simulink library "Nordic32_Lib"  (R2020b)
settings: Solver=VariableStepAuto  StartTime=0.0  StopTime=10.0  RelTol=1e-3
undefined symbols (not defined in the file or in its folder): D1, data_NREL, Delta, DiscIntNeverNeededParam, exc_Efmax, exc_Efmin, exc_Ka, exc_Ta, exc_Tb, exc_Tc, ExcData, fn, gcbh, gen_Xt, GenData, Gwind, Gwind_speed, lines, loads, mac_con, PSSData, sps_rtmsupport, time_activate_wind, trafos, wind_turbines
libraries: powerlib x18, $bdroot x13, powerlib_meascontrol x4, simulink x3, sps_avr x2, dspsigops x2, spsExcitationSystemModel x1, eeGeneralControl x1
(part 1 of 2)
settings Model: Creator=joakbj  LastModifiedBy=joakim
settings DataIOCC: ReturnWorkspaceOutputs=off
settings DebuggingCC: ArithmeticOperatorsInVariantConditions=warning
settings SFSimCC: SimUseLocalCustomCode=off  CustomCodeUndefinedFunction=UseInterfaceOnly
settings RTWCC: RTWUseLocalCustomCode=off
settings CodeAppCC: StateflowObjectComments=on

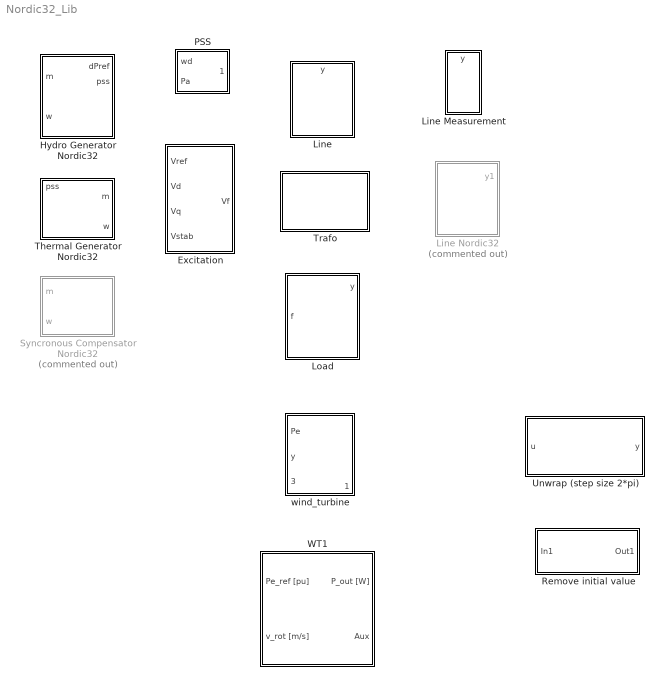
== system Nordic32_Lib ==
  Excitation : Subsystem  mask{K_a=300, sat_bounds=[0, 5]}
      mask prompts: K_a "gain"; sat_bounds "Saturation"
  Hydro Generator Nordic32 : Subsystem  mask{i=1, gen_data=GenData, pss_data=PSSData, exc_data=ExcData, ii=1, FCR_reg=tf(1), fn=fn, open_loop_on=0}
      mask prompts: i "Generator Number"; gen_data "Generator and Governor Data Table"; pss_data "PSS Data Table"; exc_data "Exciter Data Table"; ii "FCR regulator number"; FCR_reg "FCR controller transfer function"; fn "Nominal Frequency"; open_loop_on "Open loop test?"
      mask init:
      | % GenNumber = i;
      | gen_data = gen_data(i,:);
      | pss_data = pss_data(i,:);
      | exc_data = exc_data(i,:);
      | 
      | % Name to display
      | if gen_data.GenType == 1;
      |     if gen_data.GovType == 1;
      |         name = ['Hydro G', num2str(i)]; % Salient pole generator with hydro governor
      |         % Governor parameters
      |         gov_Ta = gen_data.Ta;
      |         % Gate opening limits [gmin, gmax (pu)  vgmin,vgmax(pu/s)]
      |         gov_gate= [gen_data.gMIN,  gen_data.gMAX,...
      |                   -gen_data.vgMAX, gen_data.vgMAX];
      |         % Permanent droop and regular [Rp Kp Ki Kd Td] %%% UNUSED
      | %         gov_gain = [gen_data.R, 1/gen_data.r,...
      | %                     1/(gen_data.r*gen_data.Tr),...
      | %                     0/(gen_data.r), gen_data.Tf]; 
      |         gov_num = FCR_reg.NUM{1}; % Replaces gov_gain
      |         gov_den = FCR_reg.DEN{1};
      |         gov_TW = gen_data.TW;        
      |     else
      |         name = ['erSCG', num2str(i)]; % Salient pole syncronous compensator
      |     end
      | elseif gen_data.GenType == 2;
      |     if gen_data.GovType == 0;
      |         name = ['erTG', num2str(i)]; % Round rotor generator, thermal plan no governor
      |     else
      |         name = ['erTgovG', num2str(i)]; % No Round rotor generator should have governor
      |     end
      | end
      | 
      | P = gen_data.PGEN;
      | Qmin = gen_data.QMIN;
      | Qmax = gen_data.QMAX;
      | Sb = gen_data.MBASE;
      | 
      | %% Display set power, need to adjust character length
      | set_power = ['P ', num2str(round(P,0))];
      | base_power = ['Sb ', num2str(round(Sb,0))];
      | fcr_name = ['FCR ', num2str(ii)];
      | l1 = strlength(name);
      | l2 = strlength(set_power);
      | l3 = strlength(base_power);
      | l4 = strlength(fcr_name);
      | lmax = max([l1,l2,l3,l4]);
      | 
      | for iter = 1:lmax-l1 % 
      |     name = [name, ' '];
      | end
      | for iter = 1:lmax-l2 % String with generator name has more characters
      |     set_power = [set_power, ' '];
      | end
      | for iter = 1:lmax-l3 % String with generator name has more characters
      |     base_power = [base_power, ' '];
      | end
      | for iter = 1:lmax-l4 % String with generator name has more characters
      |     fcr_name = [fcr_name, ' '];
      | end
      | 
      | name = [name;set_power;base_power;fcr_name];
      | 
      | % Generator parameters
      | gen_Pn = gen_data.MBASE; % Nominal power (MW)
      | gen_Vn = gen_data.BSKV; % Nominal voltage (kV)
      | % Reactances [Xd Xd' Xd'' Xq Xq'' Xl] (pu)
      | gen_X = [gen_data.Xd, gen_data.Xdp, gen_data.Xdpp,...
      |      gen_data.Xq, gen_data.Xqpp, gen_data.XL];
      | % Time constants [Tdo' Tdo'' Tqo''] (s)
      | gen_T = [gen_data.Td0p, gen_data.Td0pp, gen_data.Tq0pp];
      | gen_H = gen_data.H; % Inertia coefficient (s)
      | 
      | %% Governor Secondary (Frequency restoration)
      | % Ri = gen_data.Ri;
      | % Generator trafo (H)
      | % gen_Xt = gen_data.Xt*gen_Vn/(gen_Pn*2*pi*fn);
      | 
      | % gen_X = gen_X + gen_data.Xt;
      mask Display: disp(name)
  Line : Subsystem  mask{i=1, data=lines, fn=fn}
      mask prompts: i "Line Number"; data "Line Data Table"; fn "Nominal Freq"
      mask init:
      | km = data.km(i);
      | Vn = data.V(i);
      settings: PortSchema="{\"entries\":[{\"content\":{\"sides\":[{\"content\":{\"connectorIds\":[\"LConn1\",\"LConn2\",\"LConn3\"]},\"type\":\"ConnectorPlacement.EquallySpacedRectSide\",\"uuid\":\"159cc543-018e-4826-b622-a4d07c97e386\"},{\"content\":{\"connectorIds\":[\"RConn1\",\"RConn2\",\"RConn3\"],\"side\":\"RIGHT\"},\"type\":\"ConnectorPlacement.EquallySpacedRectSide\",\"uuid\":\"cb1aeae8-69bb-45ac-8689-4e8674d58501\"},{\"content\":{\"connectorIds\":[\"Out1\"],\"side\":\"TOP\"},\"type\":\"ConnectorPlacement.EquallySpacedRectSide\",\"uuid\":\"62a962af-3de7-4ff9-a859-7af1186eef9e\"}]},\"type\":\"ConnectorPlacement.EquallySpacedConnector\",\"uuid\":\"81b99b7d-1491-4204-9648-8ec0c780f157\"}],\"packageUris\":[\"http://schema.mathworks.com/mf0/Connector/19700101\"],\"version\":\"1.0\"}"
      mask Display:
      | str1 = [num2str(i)];
      | % str1 = [num2str(i)];
      | str2 = [num2str(data.from(i))];
      | str3 = [num2str(data.to(i))];
      | str4 = [num2str(data.km(i)) 'km'];
      | 
      | 
      | m = max([length(str1), length(str2), length(str3),...
      |     length(str4)]);
      | 
      | for j = length(str1):m-1
      |     str1 = [str1, ' '];
      | end
      | for j = length(str2):m-1
      |     str2 = [str2, ' '];
      | end
      | for j = length(str3):m-1
      |     str3 = [str3, ' '];
      | end
      | for j = length(str4):m-1
      |     str4 = [str4, ' '];
      | end
      | 
      | 
      | disp([str1; str2; str3; str4])
  Line Measurement : Subsystem
      settings: PortSchema="{\"entries\":[{\"content\":{\"sides\":[{\"content\":{\"connectorIds\":[\"LConn1\",\"LConn2\",\"LConn3\"]},\"type\":\"ConnectorPlacement.EquallySpacedRectSide\",\"uuid\":\"159cc543-018e-4826-b622-a4d07c97e386\"},{\"content\":{\"connectorIds\":[\"RConn1\",\"RConn2\",\"RConn3\"],\"side\":\"RIGHT\"},\"type\":\"ConnectorPlacement.EquallySpacedRectSide\",\"uuid\":\"cb1aeae8-69bb-45ac-8689-4e8674d58501\"},{\"content\":{\"connectorIds\":[\"Out1\"],\"side\":\"TOP\"},\"type\":\"ConnectorPlacement.EquallySpacedRectSide\",\"uuid\":\"62a962af-3de7-4ff9-a859-7af1186eef9e\"}]},\"type\":\"ConnectorPlacement.EquallySpacedConnector\",\"uuid\":\"81b99b7d-1491-4204-9648-8ec0c780f157\"}],\"packageUris\":[\"http://schema.mathworks.com/mf0/Connector/19700101\"],\"version\":\"1.0\"}"
      mask Display: disp(['|V|'; 'ang'; ' P '; ' Q '])
  Line Nordic32 : Subsystem  Commented=on  mask{i=1, data=lines, fn=fn}
      mask prompts: i "Line Number"; data "Line Data Table"; fn "Nominal frequency"
      mask init:
      | r = data.r(i);
      | r0 = data.r0(i);
      | l = data.l(i);
      | l0 = data.l0(i);
      | c = data.c(i);
      | c0 = data.c0(i);
      | Vn = data.V(i);
      mask Display: disp([i;data.from(i);data.to(i)])
  Load : Subsystem  mask{i=1, data=loads, fn=fn, local_freq=1}
      mask prompts: i "Load numer"; data "Load Data Table"; fn "Nominal Frequency"; local_freq "Use local frequency for loads"
      mask init:
      | data_ = data(i,:);
      | BUS = data_.BUS;
      | Vn = data_.V;
      | PL = data_.PL;
      | PL_freq = data_.PL_freq;
      | QL = data_.QL;
      | np = data_.np;
      | nq = data_.nq;
      | PSHUNT = data_.PSHUNT;
      | QSHUNT = data_.QSHUNT; % Capacitor (Negative means reactor)
      | if QSHUNT < 0
      |     QSHUNTpos = 0;
      |     QSHUNTneg = -QSHUNT;
      | else
      |     QSHUNTpos = QSHUNT;
      |     QSHUNTneg = 0;
      | end
      | 
      | %% Display active load, need to adjust character length
      | name = [num2str(BUS)];
      | strPL = ['PL ', num2str(PL)];
      | strQL = ['QL ', num2str(QL)];
      | strSH= ['SH ', num2str(QSHUNT)];
      | strV= [num2str(Vn), ' kV'];
      | l1 = strlength(name);
      | l2 = strlength(strPL);
      | l3 = strlength(strQL);
      | l4 = strlength(strSH);
      | l5 = strlength(strV);
      | lmax = max([l1,l2,l3,l4,l5]);
      | 
      | if lmax > l1
      | for iter = 1:lmax-l1 % String with set power has more characters
      |     name = [name, ' '];
      | end
      | end
      | if lmax >l2
      | for iter = 1:lmax-l2 % String with generator name has more characters
      |     strPL = [strPL, ' '];
      | end
      | end
      | if lmax > l3
      | for iter = 1:lmax-l3 % String with generator name has more characters
      |     strQL = [strQL, ' '];
      | end
      | end
      | if lmax > l4
      | for iter = 1:lmax-l4 % String with generator name has more characters
      |     strSH = [strSH, ' '];
      | end
      | end
      | if lmax > l5
      | for iter = 1:lmax-l5 % String with generator name has more characters
      |     strV = [strV, ' '];
      | end
      | end
      | 
      | name = [name;strPL;strQL;strSH;strV];
      mask Display: disp([name])
  "PSS " : Subsystem  mask(Power System Stabilizer, Nordic32){Tpss=[0, 0, 0, 0], Kpss=0, sat_bounds=[-0.05, 0.05], Tw=4.5, Tf=0.05}
      mask prompts: Tpss "time constants [T1, T2, T3, T4]"; Kpss "gain"; sat_bounds "saturation"; Tw "washout"; Tf "low_pass"
      mask help: This block implements a Power System Stabilizer as defined in Nordic32 CIGRE report
      mask init:
      | T1 = Tpss(1);
      | T2 = Tpss(2);
      | T3 = Tpss(3);
      | T4 = Tpss(4);
      | VMIN = sat_bounds(1);
      | VMAX = sat_bounds(2);
  Remove initial value : Subsystem
  Syncronous Compensator Nordic32 : Subsystem  Commented=on  mask{i=13, gen_data=GenData, pss_data=PSSData, exc_data=ExcData, fn=fn}
      mask prompts: i "Generator Number"; gen_data "Generator and Governor Data Table"; pss_data "PSS Data Table"; exc_data "Exciter Data Table"; fn "Nominal Frequency"
      mask init:
      | % GenNumber = i;
      | gen_data = gen_data(i,:);
      | pss_data = pss_data(i,:);
      | exc_data = exc_data(i,:);
      | 
      | % Name to display
      | if gen_data.GenType == 1;
      |     if gen_data.GovType == 1;
      |         name = ['erHgovG', num2str(i)]; % Salient pole generator with hydro governor
      |         % Governor parameters
      |         gov_Ta = gen_data.Ta;
      |         % Gate opening limits [gmin, gmax (pu)  vgmin,vgmax(pu/s)]
      |         gov_gate= [gen_data.gMIN,  gen_data.gMAX,...
      |                   -gen_data.vgMAX, gen_data.vgMAX];
      |         % Permanent droop and regular [Rp Kp Ki Kd Td]
      |         gov_gain = [gen_data.R, 1/gen_data.r,...
      |                     1/(gen_data.r*gen_data.Tr),...
      |                     0, gen_data.Tf];
      |         gov_TW = gen_data.TW;        
      |     else
      |         name = ['SCG', num2str(i)]; % Salient pole syncronous compensator
      |     end
      | elseif gen_data.GenType == 2;
      |     if gen_data.GovType == 0;
      |         name = ['erTG', num2str(i)]; % Round rotor generator, thermal plan no governor
      |     else
      |         name = ['erTgovG', num2str(i)]; % No Round rotor generator should have governor
      |     end
      | end
      | 
      | P = gen_data.PGEN;
      | Qmin = gen_data.QMIN;
      | Qmax = gen_data.QMAX;
      | Sb = gen_data.MBASE;
      | 
      | %% Display set power, need to adjust character length
      | set_power = ['P ', num2str(P)];
      | base_power = ['Sb ', num2str(Sb)];
      | l1 = strlength(name);
      | l2 = strlength(set_power);
      | l3 = strlength(base_power);
      | lmax = max([l1,l2,l3]);
      | 
      | for iter = 1:lmax-l1 % 
      |     name = [name, ' '];
      | end
      | for iter = 1:lmax-l2 % String with generator name has more characters
      |     set_power = [set_power, ' '];
      | end
      | for iter = 1:lmax-l3 % String with generator name has more characters
      |     base_power = [base_power, ' '];
      | end
      | 
      | name = [name;set_power;base_power];
      | 
      | % Generator parameters
      | gen_Pn = gen_data.MBASE; % Nominal power (MW)
      | gen_Vn = gen_data.BSKV; % Nominal voltage (kV)
      | % Reactances [Xd Xd' Xd'' Xq Xq'' Xl] (pu)
      | gen_X = [gen_data.Xd, gen_data.Xdp, gen_data.Xdpp,...
      |      gen_data.Xq, gen_data.Xqpp, gen_data.XL];
      | % Time constants [Tdo' Tdo'' Tqo''] (s)
      | gen_T = [gen_data.Td0p, gen_data.Td0pp, gen_data.Tq0pp];
      | gen_H = gen_data.H; % Inertia coefficient (s)
      | % Generator trafo (H)
      | % gen_Xt = gen_data.Xt*gen_Vn/(gen_Pn*2*pi*fn);
      | % gen_X = gen_X + gen_data.Xt;
      | 
      | % Exciter parameters
      | exc_Ka = exc_data.K;
      | exc_Ta = exc_data.TC;
      | exc_Tb = exc_data.TAdivbyTB*exc_data.TB;
      | exc_Tc = exc_data.TB;
      | exc_Efmin = exc_data.MIN;
      | exc_Efmax = exc_data.MAX;
      | 
      | % PSS
      | PSSNumber = pss_data.PSSNumber;
      mask Display: disp(name)
  Thermal Generator Nordic32 : Subsystem  mask{i=4, gen_data=GenData, pss_data=PSSData, exc_data=ExcData, fn=fn}
      mask prompts: i "Generator Number"; gen_data "Generator and Governor Data Table"; pss_data "PSS Data Table"; exc_data "Exciter Data Table"; fn "Nominal Frequency"
      mask init:
      | % GenNumber = i;
      | gen_data = gen_data(i,:);
      | pss_data = pss_data(i,:);
      | exc_data = exc_data(i,:);
      | 
      | % Name to display
      | if gen_data.GenType == 1;
      |     if gen_data.GovType == 1;
      |          name = ['erHgovG', num2str(i)]; % Salient pole generator with hydro governor
      | %         Governor parameters
      | %         gov_Ta = gen_data.Ta;
      | %         Gate opening limits [gmin, gmax (pu)  vgmin,vgmax(pu/s)]
      | %         gov_gate= [gen_data.gMIN,  gen_data.gMAX,...
      | %                   -gen_data.vgMAX, gen_data.vgMAX];
      | %         Permanent droop and regular [Rp Kp Ki Kd Td]
      | %         gov_gain = [gen_data.R, 1/gen_data.r,...
      | %                     1/(gen_data.r*gen_data.Tr),...
      | %                     0, gen_data.Tf];
      | %         gov_TW = gen_data.TW;        
      |     else
      |         name = ['erSCG', num2str(i)]; % Salient pole syncronous compensator
      |     end
      | elseif gen_data.GenType == 2;
      |     if gen_data.GovType == 0;
      |         name = ['Th G', num2str(i)]; % Round rotor generator, thermal plan no governor
      |     else
      |         name = ['erTgovG', num2str(i)]; % No Round rotor generator should have governor
      |     end
      | end
      | 
      | P = gen_data.PGEN;
      | Qmin = gen_data.QMIN;
      | Qmax = gen_data.QMAX;
      | Sb = gen_data.MBASE;
      | 
      | %% Display set power, need to adjust character length
      | set_power = ['P ', num2str(round(P,0))];
      | base_power = ['Sb ', num2str(round(Sb,0))];
      | l1 = strlength(name);
      | l2 = strlength(set_power);
      | l3 = strlength(base_power);
      | lmax = max([l1,l2,l3]);
      | 
      | for iter = 1:lmax-l1 % 
      |     name = [name, ' '];
      | end
      | for iter = 1:lmax-l2 % String with generator name has more characters
      |     set_power = [set_power, ' '];
      | end
      | for iter = 1:lmax-l3 % String with generator name has more characters
      |     base_power = [base_power, ' '];
      | end
      | 
      | name = [name;set_power;base_power];
      | 
      | % Generator parameters
      | gen_Pn = gen_data.MBASE; % Nominal power (MW)
      | gen_Vn = gen_data.BSKV; % Nominal voltage (kV)
      | % Reactances [Xd Xd' Xd'' Xq Xq' Xq'' Xl] (pu)
      | gen_X = [gen_data.Xd, gen_data.Xdp, gen_data.Xdpp,...
      |          gen_data.Xq, gen_data.Xqp, gen_data.Xqpp, gen_data.XL];
      | % Time constants [Tdo' Tdo'' Tqo' Tqo''] (s)
      | gen_T = [gen_data.Td0p, gen_data.Td0pp,...
      |          gen_data.Tq0p, gen_data.Tq0pp];
      | gen_H = gen_data.H; % Inertia coefficient (s)
      | % Generator trafo (H)
      | gen_Xt = gen_data.Xt*gen_Vn/(gen_Pn*2*pi*fn);
      | % gen_X = gen_X + gen_data.Xt;
      mask Display: disp(name)
  Trafo : Subsystem  mask{i=2, data=trafos, fn=fn}
      mask prompts: i "Trafo number"; data "Trafo Data Table"; fn "Nominal frequency"
      mask init:
      | V1 = data.V1(i);
      | V2 = data.V2(i);
      | L2 = data.L2(i);
      | ratio = data.ratio(i);
      | Sbase = data.Sbase(i);
      mask Display:
      | str1 = [num2str(i)];
      | % str1 = [num2str(i)];
      | str2 = [num2str(data.from(i)), ': ', num2str(data.V1(i)), 'kV'];
      | str3 = [num2str(data.to(i)), ': ', num2str(data.V2(i)), 'kV'];
      | str4 = ['x=',  num2str(data.L2(i)) 'pu'];
      | str5 = ['Sb=', num2str(data.Sbase(i))];
      | 
      | m = max([length(str1), length(str2), length(str3),...
      |     length(str4),length(str5)]);
      | 
      | for j = length(str1):m-1
      |     str1 = [str1, ' '];
      | end
      | for j = length(str2):m-1
      |     str2 = [str2, ' '];
      | end
      | for j = length(str3):m-1
      |     str3 = [str3, ' '];
      | end
      | for j = length(str4):m-1
      |     str4 = [str4, ' '];
      | end
      | for j = length(str5):m-1
      |     str5 = [str5, ' '];
      | end
      | 
      | disp([str1; str2; str3; str4; str5])
  Unwrap (step size 2*pi) : Subsystem
  WT1 : Subsystem  mask(Wind Turbine){w_gen_ini=data_NREL.w_initial, beta_ini=0, auto=off, torq_ini=data_NREL.torque_initial, data=data_NREL}
      mask prompts: w_gen_ini "Initial generator velocity  [rad/s]"; beta_ini "Initial blade pitch [degrees]"; auto "Auto initial torque"; torq_ini "Initial generator torque"; data "Data NREL Wind turbine"
      mask help: NREL 5MW Virtual Turbine
      mask init:
      | %l=load(file);
      | env=data.env;
      | wt=data.wt;
      | wt.ctrl.gen.ini=w_gen_ini;
      | ctrl=data.ctrl;
      | 
      | if(auto)
      |     wt.ctrl.torq.ini=min(interp1(wt.ctrl.torq.wg,wt.ctrl.torq.M,w_gen_ini,'spline'),wt.ctrl.torq.lim);
      | else
      |     wt.ctrl.torq.ini=torq_ini;
      | end
      | 
      | wt.pitch.ini=beta_ini;
      | wt.ctrl.pitch.ini=beta_ini;
      | wt.gen.torq.ini=wt.ctrl.torq.ini;
      | wt.gen.ini=w_gen_ini;
      | wt.rotor.ini=w_gen_ini/wt.gen.N;
      mask Display:
      | image(imread('NREL.png'))
      | 
      | port_label('output',1,'P [W]')
      | % port_label('output',2,'CT')
      | % port_label('output',3,'w_gen [rad/s]')
      | % port_label('output',4,'v_nac [m/s]')
      | % port_label('output',5,'pitch [deg]')
      | % port_label('output',6,'M_shaft [Nm]')
      | % port_label('output',7,'M_tow [Nm]')
      | % port_label('output',8,'Aux')
      | port_label('output',2,'Aux')
      | 
      | port_label('input',1,'P/P_opt [pu]')
      | port_label('input',2,'v_rot [m/s]')
      | % port_label('input',3,'v_nac [m/s]')
  wind_turbine : Subsystem  mask{i=1, data=wind_turbines, data_NREL=data_NREL, fn=fn, time_activate_wind=time_activate_wind, Gwind=Gwind, Gwind_speed=Gwind_speed, FCR=tf(1)}
      mask prompts: i "Turbine number"; data "Wind Turbine Load Flow Data"; data_NREL "Wind Model Data"; fn "Nominal freqeuncy"; time_activate_wind "Activate wind turbine model at time:"; Gwind "Linear model, Pref -> Pe"; Gwind_speed "Linear model, Pref -> speed"; FCR "FCR, y -> Pref"
      mask init:
      | data = data(i,:); 
      | 
      | Vn = data.BSKV;
      | MBASE = data.MBASE;
      | POPT = data.POPT;
      | 
      | if iscell(data_NREL)
      |     data_NREL = data_NREL{i};
      | end
      | 
      | strWindSpeed = ['v = ', num2str(data.V_WIND)];
      | strWind = ['wind(',num2str(i),') ' num2str(MBASE)];
      | strWindOpt = ['Popt ', num2str(round(POPT,0))];
      | strV= [num2str(Vn), ' kV'];
      | 
      | l1 = strlength(strWind);
      | l2 = strlength(strWindOpt);
      | l3 = strlength(strV);
      | l4 = strlength(strWindSpeed);
      | lmax = max([l1,l2,l3,l4]);
      | 
      | if lmax > l1
      | for iter = 1:lmax-l1 % String with generator name has more characters
      |     strWind = [strWind, ' '];
      | end
      | end
      | if lmax > l2
      | for iter = 1:lmax-l2 % String with generator name has more characters
      |     strWindOpt = [strWindOpt, ' '];
      | end
      | end
      | if lmax > l3
      | for iter = 1:lmax-l3 % String with generator name has more characters
      |     strV = [strV, ' '];
      | end
      | end
      | if lmax > l4
      | for iter = 1:lmax-l4 % String with generator name has more characters
      |     strWindSpeed = [strWindSpeed, ' '];
      | end
      | end
      | 
      | name = [strWindSpeed;strWind;strWindOpt;strV];
      settings: PortSchema="{\"entries\":[{\"content\":{\"sides\":[{\"content\":{\"connectorIds\":[\"LConn1\",\"LConn2\",\"LConn3\",\"In1\"]},\"type\":\"ConnectorPlacement.EquallySpacedRectSide\",\"uuid\":\"48445341-a685-4506-9ec8-e376e0c1b939\"},{\"content\":{\"connectorIds\":[\"Out1\",\"Out2\",\"Out3\"],\"side\":\"RIGHT\"},\"type\":\"ConnectorPlacement.EquallySpacedRectSide\",\"uuid\":\"cf3481ef-9523-4ae9-af94-5a03f7da080c\"},{\"content\":{\"connectorIds\":[],\"side\":\"TOP\"},\"type\":\"ConnectorPlacement.EquallySpacedRectSide\",\"uuid\":\"cf4caa18-6df0-400d-a59e-8b335f5a193c\"}]},\"type\":\"ConnectorPlacement.EquallySpacedConnector\",\"uuid\":\"872d10b1-fdd8-4789-878b-9f44ab3824be\"}],\"packageUris\":[\"http://schema.mathworks.com/mf0/Connector/19700101\"],\"version\":\"1.0\"}"
      mask Display: disp([name])

== system Nordic32_Lib/Excitation ==
  Vref : Inport
  Vd : Inport  Port=2
  Vq : Inport  Port=3
  Vstab : Inport  Port=4
  EXCITATION Nordic32 : sps_avr/Excitation System  Commented=on  tr=0.02  reg=[exc_Ka, exc_Ta]  exc=[ 1, 0 ]  tgr=[exc_Tb, exc_Tc]  damp=[ 1e-3 0.1]*0  sat=[ 0, 0 ]  lim=[exc_Efmin, exc_Efmax, 0 ]  v0=[1,1.07168]
      settings: SourceProductBaseCode=PS
  Excitation Standard : Subsystem  DialogController=POWERSYS.PowerSysDialog  LoadFcn=sps_rtmsupport('LoadFcn', gcbh);  StartFcn=sps_rtmsupport('StartFcn', gcbh);  StopFcn=sps_rtmsupport('StopFcn', gcbh);  mask(Excitation System){tr=20e-3, reg=[ K_a, 0.001 ], exc=[ 1, 0 ], tgr=[ 0, 0 ], damp=[ 0.001, 0.1 ], sat=[ 0, 0 ], lim=[sat_bounds(1), sat_bounds(2), 0 ], v0=[1.0  1.28]}
      mask prompts: tr "Low-pass filter time constant Tr(s):"; reg "Regulator gain and time constant [ Ka()  Ta(s) ]:"; exc "Exciter  [ Ke()  Te(s) ]:"; tgr "Transient gain reduction [ Tb(s)  Tc(s) ]:"; damp "Damping filter gain and time constant  [ Kf()  Tf(s)  ]:"; sat "Field saturation parameters [ A, B ]:"; lim "Regulator output limits and gain [ Efmin, Efmax (pu), Kp() ]:"; v0 "Initial values of terminal voltage  and field voltage [ Vt0 (pu) Vf0(pu) ] :"
      mask help:
      | Implements an IEEE type 1 synchronous machine voltage regulator combined
      | to an exciter.
      |
      | The output of the block is the field voltage vfd, in pu,  to be applied to the Vf
      | Simulink input of a Synchronous Machine block.
      |
      | Connect the Vd and Vq measurements signals of the Synchronous Machine block
      | (signals 9 and 10)  to  the Vd and Vq inputs of the Excitation System block.
      mask init:
      | block = gcb;
      | [Ts, WantBlockChoice,MaskType, ka,ta,ke,te,tb,tc,kf,tf,efmin,efmax,kp,a,b] = powericon('ExcitationSystemInit',block,-2,reg,exc,tgr,damp,lim,sat);
      | powericon('SetInternalModels','set',block,WantBlockChoice);
      settings: CopyFcn=sps_rtmsupport('CopyFcn', gcbh);  DeleteFcn=sps_rtmsupport('DeleteFcn', gcbh);  UndoDeleteFcn=sps_rtmsupport('UndoDeleteFcn', gcbh);  ModelCloseFcn=sps_rtmsupport('ModelCloseFcn', gcbh);  PreSaveFcn=sps_rtmsupport('PreSaveFcn', gcbh);  PostSaveFcn=sps_rtmsupport('PostSaveFcn', gcbh);  NameChangeFcn=sps_rtmsupport('NameChangeFcn', gcbh);  PreCopyFcn=sps_rtmsupport('PreCopyFcn', gcbh);  OpenFcn=sps_rtmsupport('OpenFcn', gcbh, []);  CloseFcn=sps_rtmsupport('CloseFcn', gcbh);  PreDeleteFcn=sps_rtmsupport('PreDeleteFcn', gcbh);
      mask Help: helpview(psbhelp);
      mask Display: disp('')
  Vf : Outport
  wires:
  Excitation Standard/1(Vf) -> Vf/1
  Vq/1 -> Excitation Standard/3(Vq)
  Vd/1 -> Excitation Standard/2(Vd)
  Vstab/1 -> Excitation Standard/4(Vstab)
  Vref/1 -> Excitation Standard/1(Vref)

== system Nordic32_Lib/Hydro Generator Nordic32 ==
  dPref : Inport
  pss : Inport  Port=2
  " MBASE MVA 400 kV-400 kV" : powerlib/Elements/Three-Phase Transformer (Two Windings)  Winding1Connection=Delta (D1)  Winding2Connection=Yg  CoreType=Three single-phase transformers  SetSaturation=off  Hysteresis=off  DataFile='hysteresis'  SetInitialFlux=off  Measurements=None  UNITS=pu  NominalPower="[ gen_Pn*1e6  fn ]"  Winding1="[ gen_Vn*1e3  1e-6   0  ]"  Winding2="[ gen_Vn*1e3   1e-6  gen_data.Xt ]"  Rm=500  Lm=500  L0=0.5  Saturation="[ 0,0  ;  0.005,1.2  ;  1.0,1.4 ]"  InitialFluxes=[ 0.8 , -0.8 , 0.7 ]  BreakLoop=off  DiscreteSolver=Trapezoidal iterative  DataType=off  TransfoNumber=0
  Bus Selector : BusSelector  OutputSignals="Rotor speed  wm  (pu)"
  Generator : powerlib/Machines/Synchronous Machine pu Standard  PresetModel=No  MechanicalLoad=Mechanical power Pm  ShowDetailedParameters=on  RotorType=Salient-pole  Units=per unit standard parameters  MeasurementBus=off  NominalParameters=[gen_Pn*1e6, gen_Vn*1e3, fn]  Reactances1="[mac_con(1,6:8)  mac_con(1,11:13)  mac_con(1,4)]"  Reactances2=gen_X  dAxisTimeConstants=Open-circuit  qAxisTimeConstants=Open-circuit  TimeConstants1=gen_T  TimeConstants2="[mac_con(1,9:10)  mac_con(1,14:15)]"  TimeConstants3=[]  TimeConstants4=[]  TimeConstants5=[ 1.01, 0.053, 0.1 ]  TimeConstants6=[]  TimeConstants7=gen_T  TimeConstants8=[]  StatorResistance=[1e-9]  Mechanical="[gen_H 0  4]"  PolePairs=4  InitialConditions=[0 -53.3817 1.03438 1.03438 1.03438 11.5505 -108.45 131.55 1.07168]  SetSaturation=off  Saturation=[0.6404,0.7127,0.8441,0.9214,0.9956,1.082,1.19,1.316,1.457;0.7,0.7698,0.8872,0.9466,0.9969,1.046,1.1,1.151,1.201]  LoadFlowParameters=[1 1000000000 0 0 0]  TsPowergui=0  TsBlock=-1  IterativeModel=Forward Euler  IterativeDiscreteModel=Trapezoidal non iterative  BusType=PV  Pref=P*1e6  Qref=0  Qmin=Qmin*1e6  Qmax=Qmax*1e6  PLF=0  QLF=0
      settings: AttributesFormatString=\n\n
  Pref : Constant
  Turbine & Regulators : Subsystem
  Vref : Constant
  A : PMIOPort  Side=Left
  B : PMIOPort  Port=2  Side=Left
  C : PMIOPort  Port=3  Side=Left
  m : Outport  VectorParamsAs1DForOutWhenUnconnected=off
  w : Outport  Port=2  VectorParamsAs1DForOutWhenUnconnected=off
  wires:
  Turbine & Regulators/2(Vf) -> Generator/2
  Generator/1 -> Turbine & Regulators/1(m)
  Vref/1 -> Turbine & Regulators/3(Vref)
  Turbine & Regulators/3(Signals) -> m/1, Bus Selector/1
  Turbine & Regulators/1(Pm) -> Generator/1
  Pref/1 -> Turbine & Regulators/2(Pref)
  Bus Selector/1 -> w/1  "<Rotor speed  wm  (pu)>"
  dPref/1 -> Turbine & Regulators/4(open_loop)
  pss/1 -> Turbine & Regulators/5(d_Vstab)
  connections:
  " MBASE MVA 400 kV-400 kV"/LConn1 -- Generator/RConn1
  " MBASE MVA 400 kV-400 kV"/LConn2 -- Generator/RConn2
  " MBASE MVA 400 kV-400 kV"/LConn3 -- Generator/RConn3
  " MBASE MVA 400 kV-400 kV"/RConn1 -- A/RConn1
  B/RConn1 -- " MBASE MVA 400 kV-400 kV"/RConn2
  C/RConn1 -- " MBASE MVA 400 kV-400 kV"/RConn3

== system Nordic32_Lib/Line ==
  Bus Creator : BusCreator  Inputs=2
  Distributed Parameters Line : powerlib/Elements/Distributed Parameters Line  Phases=3  Length=km  Frequency=fn  Resistance=[0.01273 0.3864]  Inductance="[0.9337e-3  4.1264e-3]"  Capacitance=[12.74e-9 7.751e-9]  x1=[0 0 0 0; 0.0001244 0 0 0; 0.0002488 0 0 0; 0.0003733 0 0 0; 0.0004977 0 0 0; 0.0006221 0 0 0]  x2=[0 0 0 0; 0.0001244 0 0 0; 0.0002488 0 0 0; 0.0003733 0 0 0; 0.0004977 0 0 0; 0.0006221 0 0 0]  x3=[0 0 0 0; 0.0001244 0 0 0; 0.0002488 0 0 0; 0.0003733 0 0 0; 0.0004977 0 0 0; 0.0006221 0 0 0]  x4=[0 0 0 0; 0.0001244 0 0 0; 0.0002488 0 0 0; 0.0003733 0 0 0; 0.0004977 0 0 0; 0.0006221 0 0 0]  x5=0  V1=ones(3,3)  V2=ones(3,3)  I1=ones(3,3)  I2=ones(3,3)  nHarmo=1  Measurements=None  Decoupling=off  VsMag0=0  VrMag0=0  VsAngle0=0  VrAngle0=0  IsMag0=0  IrMag0=0  IsAngle0=0  IrAngle0=0
  Line Measurement : $bdroot/Line  Measurement  SystemSampleTime=-1  VariantActivationTime=update diagram  Latency=0  AutoFrameSizeCalculation=off
      settings: PortSchema="{\"entries\":[{\"content\":{\"sides\":[{\"content\":{\"connectorIds\":[\"LConn1\",\"LConn2\",\"LConn3\"]},\"type\":\"ConnectorPlacement.EquallySpacedRectSide\",\"uuid\":\"159cc543-018e-4826-b622-a4d07c97e386\"},{\"content\":{\"connectorIds\":[\"RConn1\",\"RConn2\",\"RConn3\"],\"side\":\"RIGHT\"},\"type\":\"ConnectorPlacement.EquallySpacedRectSide\",\"uuid\":\"cb1aeae8-69bb-45ac-8689-4e8674d58501\"},{\"content\":{\"connectorIds\":[\"Out1\"],\"side\":\"TOP\"},\"type\":\"ConnectorPlacement.EquallySpacedRectSide\",\"uuid\":\"62a962af-3de7-4ff9-a859-7af1186eef9e\"}]},\"type\":\"ConnectorPlacement.EquallySpacedConnector\",\"uuid\":\"81b99b7d-1491-4204-9648-8ec0c780f157\"}],\"packageUris\":[\"http://schema.mathworks.com/mf0/Connector/19700101\"],\"version\":\"1.0\"}"
  Line Measurement1 : $bdroot/Line  Measurement  SystemSampleTime=-1  VariantActivationTime=update diagram  Latency=0  AutoFrameSizeCalculation=off
      settings: PortSchema="{\"entries\":[{\"content\":{\"sides\":[{\"content\":{\"connectorIds\":[\"LConn1\",\"LConn2\",\"LConn3\"]},\"type\":\"ConnectorPlacement.EquallySpacedRectSide\",\"uuid\":\"159cc543-018e-4826-b622-a4d07c97e386\"},{\"content\":{\"connectorIds\":[\"RConn1\",\"RConn2\",\"RConn3\"],\"side\":\"RIGHT\"},\"type\":\"ConnectorPlacement.EquallySpacedRectSide\",\"uuid\":\"cb1aeae8-69bb-45ac-8689-4e8674d58501\"},{\"content\":{\"connectorIds\":[\"Out1\"],\"side\":\"TOP\"},\"type\":\"ConnectorPlacement.EquallySpacedRectSide\",\"uuid\":\"62a962af-3de7-4ff9-a859-7af1186eef9e\"}]},\"type\":\"ConnectorPlacement.EquallySpacedConnector\",\"uuid\":\"81b99b7d-1491-4204-9648-8ec0c780f157\"}],\"packageUris\":[\"http://schema.mathworks.com/mf0/Connector/19700101\"],\"version\":\"1.0\"}"
  A : PMIOPort  Side=Left
  B : PMIOPort  Port=2  Side=Left
  C : PMIOPort  Port=3  Side=Left
  a : PMIOPort  Port=4  Side=Right
  b : PMIOPort  Port=5  Side=Right
  c : PMIOPort  Port=6  Side=Right
  y : Outport
  wires:
  Line Measurement/1 -> Bus Creator/1
  Line Measurement1/1 -> Bus Creator/2
  Bus Creator/1 -> y/1
  connections:
  Line Measurement/LConn1 -- A/RConn1
  B/RConn1 -- Line Measurement/LConn2
  C/RConn1 -- Line Measurement/LConn3
  Distributed Parameters Line/LConn1 -- Line Measurement/RConn1
  Distributed Parameters Line/LConn2 -- Line Measurement/RConn2
  Distributed Parameters Line/LConn3 -- Line Measurement/RConn3
  Distributed Parameters Line/RConn3 -- Line Measurement1/LConn3
  Line Measurement1/RConn3 -- c/RConn1
  Line Measurement1/RConn2 -- b/RConn1
  Distributed Parameters Line/RConn2 -- Line Measurement1/LConn2
  Distributed Parameters Line/RConn1 -- Line Measurement1/LConn1
  Line Measurement1/RConn1 -- a/RConn1

== system Nordic32_Lib/Line Measurement ==
  Bus Creator : BusCreator  Inputs=4
  Gain : Gain  Gain=pi/180
  Gain1 : Gain  Gain=180/pi
  "Power (3ph, Phasor)" : powerlib_meascontrol/Measurements/Power (3ph, Phasor)
      settings: SourceProductBaseCode=PS
  Sequence Analyzer (Phasor) : powerlib_meascontrol/Measurements/Sequence Analyzer (Phasor)  seq=Positive
      settings: SourceProductBaseCode=PS
  Three-Phase V-I Measurement : powerlib/Measurements/Three-Phase V-I Measurement  VoltageMeasurement=phase-to-ground  SetLabelV=off  LabelV=Vabc  Vpu=off  VpuLL=off  CurrentMeasurement=yes  SetLabelI=off  LabelI=Iabc  Ipu=off  Pbase=1e6  Vbase=400e3  OutputType=Complex  PhasorSimulation=off  PSBequivalent=0
  Unwrap pi deg : dspsigops/Unwrap  tol=pi  InputProcessing=Columns as channels (frame based)  running=off
  A : PMIOPort  Side=Left
  B : PMIOPort  Port=2  Side=Left
  C : PMIOPort  Port=3  Side=Left
  a : PMIOPort  Port=4  Side=Right
  b : PMIOPort  Port=5  Side=Right
  c : PMIOPort  Port=6  Side=Right
  y : Outport
  wires:
  "Power (3ph, Phasor)"/2 -> Bus Creator/4  "Q"
  Three-Phase V-I Measurement/2 -> "Power (3ph, Phasor)"/2
  Three-Phase V-I Measurement/1 -> Sequence Analyzer (Phasor)/1, "Power (3ph, Phasor)"/1
  Sequence Analyzer (Phasor)/1 -> Bus Creator/1  "V"
  Unwrap pi deg/1 -> Gain1/1  "ang"
  Bus Creator/1 -> y/1
  "Power (3ph, Phasor)"/1 -> Bus Creator/3  "P"
  Sequence Analyzer (Phasor)/2 -> Gain/1  "ang"
  Gain/1 -> Unwrap pi deg/1
  Gain1/1 -> Bus Creator/2  "ang"
  connections:
  Three-Phase V-I Measurement/RConn1 -- a/RConn1
  Three-Phase V-I Measurement/LConn3 -- C/RConn1
  Three-Phase V-I Measurement/RConn3 -- c/RConn1
  Three-Phase V-I Measurement/LConn2 -- B/RConn1
  Three-Phase V-I Measurement/LConn1 -- A/RConn1
  Three-Phase V-I Measurement/RConn2 -- b/RConn1

== system Nordic32_Lib/Line Nordic32 ==
  25km Area 1 : powerlib/Elements/Three-Phase PI Section Line  LConnTagsString=a|b|c  RConnTagsString=A|B|C  Length=1  Frequency=fn  Resistances=[r r0]  Inductances=[l l0]  Capacitances=[c c0]
  Line Measurement : $bdroot/Line  Measurement  SystemSampleTime=-1  VariantActivationTime=update diagram  Latency=0  AutoFrameSizeCalculation=off
      settings: PortSchema="{\"entries\":[{\"content\":{\"sides\":[{\"content\":{\"connectorIds\":[\"LConn1\",\"LConn2\",\"LConn3\"]},\"type\":\"ConnectorPlacement.EquallySpacedRectSide\",\"uuid\":\"159cc543-018e-4826-b622-a4d07c97e386\"},{\"content\":{\"connectorIds\":[\"RConn1\",\"RConn2\",\"RConn3\"],\"side\":\"RIGHT\"},\"type\":\"ConnectorPlacement.EquallySpacedRectSide\",\"uuid\":\"cb1aeae8-69bb-45ac-8689-4e8674d58501\"},{\"content\":{\"connectorIds\":[\"Out1\"],\"side\":\"TOP\"},\"type\":\"ConnectorPlacement.EquallySpacedRectSide\",\"uuid\":\"62a962af-3de7-4ff9-a859-7af1186eef9e\"}]},\"type\":\"ConnectorPlacement.EquallySpacedConnector\",\"uuid\":\"81b99b7d-1491-4204-9648-8ec0c780f157\"}],\"packageUris\":[\"http://schema.mathworks.com/mf0/Connector/19700101\"],\"version\":\"1.0\"}"
  Line Measurement1 : $bdroot/Line  Measurement  SystemSampleTime=-1  VariantActivationTime=update diagram  Latency=0  AutoFrameSizeCalculation=off
      settings: PortSchema="{\"entries\":[{\"content\":{\"sides\":[{\"content\":{\"connectorIds\":[\"LConn1\",\"LConn2\",\"LConn3\"]},\"type\":\"ConnectorPlacement.EquallySpacedRectSide\",\"uuid\":\"159cc543-018e-4826-b622-a4d07c97e386\"},{\"content\":{\"connectorIds\":[\"RConn1\",\"RConn2\",\"RConn3\"],\"side\":\"RIGHT\"},\"type\":\"ConnectorPlacement.EquallySpacedRectSide\",\"uuid\":\"cb1aeae8-69bb-45ac-8689-4e8674d58501\"},{\"content\":{\"connectorIds\":[\"Out1\"],\"side\":\"TOP\"},\"type\":\"ConnectorPlacement.EquallySpacedRectSide\",\"uuid\":\"62a962af-3de7-4ff9-a859-7af1186eef9e\"}]},\"type\":\"ConnectorPlacement.EquallySpacedConnector\",\"uuid\":\"81b99b7d-1491-4204-9648-8ec0c780f157\"}],\"packageUris\":[\"http://schema.mathworks.com/mf0/Connector/19700101\"],\"version\":\"1.0\"}"
  A : PMIOPort  Side=Left
  a : PMIOPort  Port=2  Side=Right
  B : PMIOPort  Port=3  Side=Left
  b : PMIOPort  Port=4  Side=Right
  C : PMIOPort  Port=5  Side=Left
  c : PMIOPort  Port=6  Side=Right
  y1 : Outport
  wires:
  Line Measurement/1 -> y1/1
  connections:
  Line Measurement/LConn1 -- A/RConn1
  B/RConn1 -- Line Measurement/LConn2
  C/RConn1 -- Line Measurement/LConn3
  Line Measurement/RConn1 -- 25km Area 1/LConn1
  Line Measurement/RConn2 -- 25km Area 1/LConn2
  Line Measurement/RConn3 -- 25km Area 1/LConn3
  Line Measurement1/LConn3 -- 25km Area 1/RConn3
  Line Measurement1/RConn3 -- c/RConn1
  Line Measurement1/RConn2 -- b/RConn1
  25km Area 1/RConn2 -- Line Measurement1/LConn2
  25km Area 1/RConn1 -- Line Measurement1/LConn1
  Line Measurement1/RConn1 -- a/RConn1

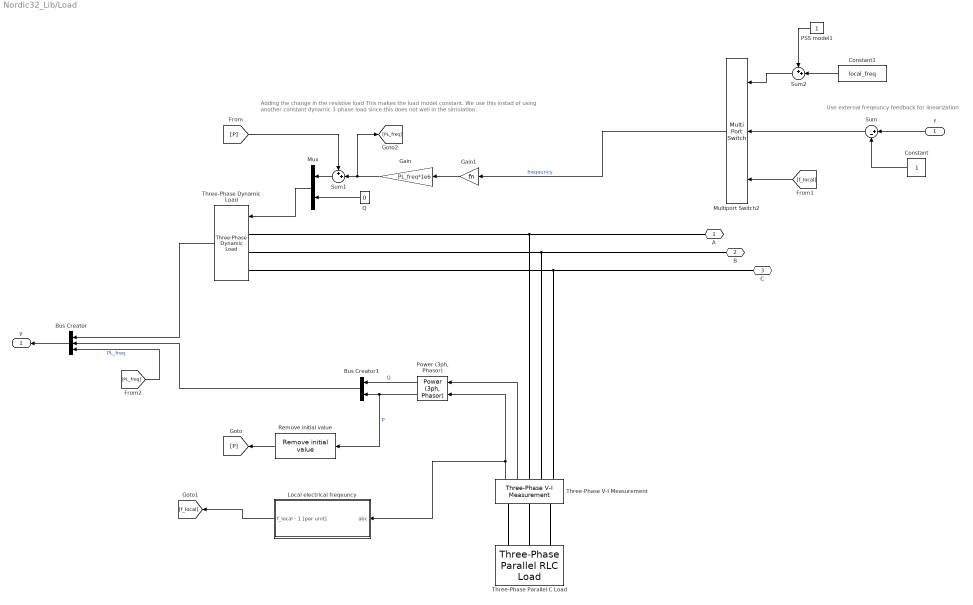
== system Nordic32_Lib/Load ==
  note: Use external freqeuncy feedback for linearization
  note: Adding the change in the resistive load
      | This makes the load model constant.
      | We use this instad of using another constant dynamic 3-phase load since this does not well in the simulation.
  f : Inport
  Bus Creator : BusCreator  Inputs=3
  Bus Creator1 : BusCreator  Inputs=2
  Constant : Constant
  Constant1 : Constant  Value=local_freq
  Gain : Gain  Gain=PL_freq*1e6
  Gain1 : Gain  Gain=fn
  Local electrical freqeuncy : Subsystem
  Multiport Switch2 : MultiPortSwitch  Inputs=2  InputSameDT=on
  Mux : Mux  Inputs=2
  PSS model1 : Constant
  "Power (3ph, Phasor)" : powerlib_meascontrol/Measurements/Power (3ph, Phasor)
      settings: SourceProductBaseCode=PS
  Q : Constant  Value=0
  Remove initial value : $bdroot/Remove initial value  SystemSampleTime=-1  VariantActivationTime=update diagram  Latency=0  AutoFrameSizeCalculation=off
  Sum : Sum  Inputs=|+-
  Sum1 : Sum  Inputs=++|
  Sum2 : Sum  Inputs=++|
  Three-Phase Dynamic Load : powerlib/Elements/Three-Phase Dynamic Load  NominalVoltage=[Vn*1e3 fn ]  ActiveReactivePowers=[0 0]  PositiveSequence=[1.001 40.526]  ExternalControl=on  NpNq=[1.3 2]  TimeConstants="[0  0  0  0]"  MinimumVoltage=0.7  Tfilter=1e-2  LoadFlowParameters=[4,0,0,0,0]
      settings: SourceProductBaseCode=PS
  Three-Phase Parallel C Load : powerlib/Elements/Three-Phase Parallel RLC Load  LConnTagsString=A|B|C  Configuration=Y (grounded)  NominalVoltage=(130000)*1.001  Vabc=[1e3 1e3 1e3]  Vabcp=[1e3 1e3 1e3]  NominalFrequency=fn  UnbalancedPower=off  ActivePower=PL*1e6+1e-6  InductivePower=(QL)*1e6+ (QSHUNTneg)*1e6  CapacitivePower=QSHUNTpos*1e6  Pabc=[10e3 9e3 11e3]  QLabc=[100 90 110]  QCabc=[100 90 110]  Pabcp=[10e3 9e3 11e3]  QLabcp=[100 90 110]  QCabcp=[100 90 110]  Measurements=None  LoadType=constant PQ
  Three-Phase V-I Measurement : powerlib/Measurements/Three-Phase V-I Measurement  VoltageMeasurement=phase-to-ground  SetLabelV=off  LabelV=Vabc  Vpu=off  VpuLL=off  CurrentMeasurement=yes  SetLabelI=off  LabelI=Iabc  Ipu=off  Pbase=100e6  Vbase=Vn*1e3  OutputType=Complex  PhasorSimulation=off  PSBequivalent=0
  A : PMIOPort  Side=Right
  B : PMIOPort  Port=2  Side=Right
  C : PMIOPort  Port=3  Side=Right
  y : Outport  VectorParamsAs1DForOutWhenUnconnected=off
  wires:
  Q/1 -> Mux/2
  Mux/1 -> Three-Phase Dynamic Load/1
  f/1 -> Sum/1
  Constant/1 -> Sum/2
  Gain1/1 -> Gain/1
  Three-Phase Dynamic Load/1 -> Bus Creator/1
  Three-Phase V-I Measurement/1 -> "Power (3ph, Phasor)"/1, Local electrical freqeuncy/1(abc)
  Local electrical freqeuncy/1(f_local - 1 [per unit]) -> [f_local]
  Three-Phase V-I Measurement/2 -> "Power (3ph, Phasor)"/2
  Bus Creator/1 -> y/1
  "Power (3ph, Phasor)"/2 -> Bus Creator1/1  "Q"
  "Power (3ph, Phasor)"/1 -> Remove initial value/1, Bus Creator1/2  "P"
  Bus Creator1/1 -> Bus Creator/2
  Remove initial value/1 -> [P]
  Sum1/1 -> Mux/1
  Gain/1 -> [PL_freq], Sum1/2
  [P] -> Sum1/1
  [PL_freq] -> Bus Creator/3  "PL_freq"
  Sum/1 -> Multiport Switch2/2
  Sum2/1 -> Multiport Switch2/1
  Constant1/1 -> Sum2/2
  PSS model1/1 -> Sum2/1
  [f_local] -> Multiport Switch2/3
  Multiport Switch2/1 -> Gain1/1  "freqeuncy"
  connections:
  A/RConn1 -- Three-Phase Dynamic Load/LConn1 -- Three-Phase V-I Measurement/RConn1
  B/RConn1 -- Three-Phase Dynamic Load/LConn2 -- Three-Phase V-I Measurement/RConn2
  C/RConn1 -- Three-Phase Dynamic Load/LConn3 -- Three-Phase V-I Measurement/RConn3
  Three-Phase Parallel C Load/LConn1 -- Three-Phase V-I Measurement/LConn1
  Three-Phase V-I Measurement/LConn2 -- Three-Phase Parallel C Load/LConn2
  Three-Phase Parallel C Load/LConn3 -- Three-Phase V-I Measurement/LConn3

== system Nordic32_Lib/PSS  ==
  wd : Inport
  Pa : Inport  Port=2
  Gain : Gain  Gain=Kpss
  Saturation : Saturate  UpperLimit=VMAX  LowerLimit=-VMIN
  Transfer Fcn : TransferFcn  Denominator=[Tf 1]
  Transfer Fcn2 : TransferFcn  Numerator=[T1 1]  Denominator=[T2 1]
  Transfer Fcn3 : TransferFcn  Numerator=[T3 1]  Denominator=[T4 1]
  Washout (Discrete or Continuous) : eeGeneralControl/Washout (Discrete or Continuous)  T=Tw  init_option=Specify as parameter  x0=0  Ts=0
      settings: SourceProductBaseCode=PS
  Vstab : Outport  VectorParamsAs1DForOutWhenUnconnected=off
  wires:
  Transfer Fcn2/1 -> Transfer Fcn3/1
  Saturation/1 -> Vstab/1
  Gain/1 -> Saturation/1
  Washout (Discrete or Continuous)/1 -> Transfer Fcn/1
  Pa/1 -> Washout (Discrete or Continuous)/1
  Transfer Fcn3/1 -> Gain/1
  Transfer Fcn/1 -> Transfer Fcn2/1

== system Nordic32_Lib/Remove initial value ==
  In1 : Inport
  Step at time 0.01 : Step  Time=0.01  Before=1  After=0  SampleTime=0
  Subsystem : Subsystem
  Sum : Sum  Inputs=-+|
  Out1 : Outport
  wires:
  Sum/1 -> Out1/1
  Subsystem/1(Out1) -> Sum/1
  Step at time 0.01/1 -> Subsystem/Enable
  In1/1 -> Sum/2, Subsystem/1(In1)

== system Nordic32_Lib/Syncronous Compensator Nordic32 ==
  Bus Selector : BusSelector  OutputSignals="Rotor speed  wm  (pu)"
  Generator : powerlib/Machines/Synchronous Machine pu Standard  PresetModel=No  MechanicalLoad=Mechanical power Pm  ShowDetailedParameters=on  RotorType=Salient-pole  Units=per unit standard parameters  MeasurementBus=off  NominalParameters=[gen_Pn*1e6, gen_Vn*1e3, fn]  Reactances1="[mac_con(1,6:8)  mac_con(1,11:13)  mac_con(1,4)]"  Reactances2=gen_X  dAxisTimeConstants=Open-circuit  qAxisTimeConstants=Open-circuit  TimeConstants1=gen_T  TimeConstants2="[mac_con(1,9:10)  mac_con(1,14:15)]"  TimeConstants3=[]  TimeConstants4=[]  TimeConstants5=[ 1.01, 0.053, 0.1 ]  TimeConstants6=[]  TimeConstants7=gen_T  TimeConstants8=[]  StatorResistance=[1e-9]  Mechanical=[gen_H 0 4]  PolePairs=4  InitialConditions=[0 -53.3817 1.03438 1.03438 1.03438 11.5505 -108.45 131.55 1.07168]  SetSaturation=off  Saturation=[0.6404,0.7127,0.8441,0.9214,0.9956,1.082,1.19,1.316,1.457;0.7,0.7698,0.8872,0.9466,0.9969,1.046,1.1,1.151,1.201]  LoadFlowParameters=[1 1000000000 0 0 0]  TsPowergui=0  TsBlock=-1  IterativeModel=Forward Euler  IterativeDiscreteModel=Trapezoidal non iterative  BusType=PV  Pref=P*1e6  Qref=0  Qmin=Qmin*1e6  Qmax=Qmax*1e6  PLF=0  QLF=0
      settings: AttributesFormatString=\n\n
  PSS model : Constant  Value=0
  Pref : Constant
  Turbine & Regulators : Subsystem
  Vref : Constant
  A : PMIOPort  Side=Left
  B : PMIOPort  Port=2  Side=Left
  C : PMIOPort  Port=3  Side=Left
  m : Outport  VectorParamsAs1DForOutWhenUnconnected=off
  w : Outport  Port=2  VectorParamsAs1DForOutWhenUnconnected=off
  wires:
  Pref/1 -> Turbine & Regulators/2(Pref)
  PSS model/1 -> Turbine & Regulators/4(PSS)
  Turbine & Regulators/2(Vf) -> Generator/2
  Generator/1 -> Turbine & Regulators/1(m)
  Vref/1 -> Turbine & Regulators/3(Vref)
  Turbine & Regulators/3(Signals) -> Bus Selector/1, m/1
  Turbine & Regulators/1(Pm) -> Generator/1
  Bus Selector/1 -> w/1  "<Rotor speed  wm  (pu)>"
  connections:
  Generator/RConn1 -- A/RConn1
  Generator/RConn2 -- B/RConn1
  Generator/RConn3 -- C/RConn1

== system Nordic32_Lib/Thermal Generator Nordic32 ==
  pss : Inport
  " MBASE MVA 400 kV-400 kV" : powerlib/Elements/Three-Phase Transformer (Two Windings)  Winding1Connection=Delta (D1)  Winding2Connection=Yg  CoreType=Three single-phase transformers  SetSaturation=off  Hysteresis=off  DataFile='hysteresis'  SetInitialFlux=off  Measurements=None  UNITS=pu  NominalPower="[ gen_Pn*1e6  fn ]"  Winding1="[ gen_Vn*1e3  1e-6   0  ]"  Winding2="[ gen_Vn*1e3   1e-6   gen_data.Xt ]"  Rm=500  Lm=500  L0=0.5  Saturation="[ 0,0  ;  0.005,1.2  ;  1.0,1.4 ]"  InitialFluxes=[ 0.8 , -0.8 , 0.7 ]  BreakLoop=off  DiscreteSolver=Trapezoidal iterative  DataType=off  TransfoNumber=0
  Bus Selector : BusSelector  OutputSignals="Rotor speed  wm  (pu)"
  Generator : powerlib/Machines/Synchronous Machine pu Standard  PresetModel=No  MechanicalLoad=Mechanical power Pm  ShowDetailedParameters=on  RotorType=Round  Units=per unit standard parameters  MeasurementBus=off  NominalParameters=[gen_Pn*1e6, gen_Vn*1e3, fn]  Reactances1=gen_X  Reactances2=gen_X  dAxisTimeConstants=Open-circuit  qAxisTimeConstants=Open-circuit  TimeConstants1=gen_T  TimeConstants2=gen_T  TimeConstants3=[]  TimeConstants4=[]  TimeConstants5=[ 1.01, 0.053, 0.1 ]  TimeConstants6=[]  TimeConstants7=[]  TimeConstants8=gen_T  StatorResistance=[1e-9]  Mechanical=[gen_H 0 4]  PolePairs=4  InitialConditions=[0 -53.3817 1.03438 1.03438 1.03438 11.5505 -108.45 131.55 1.07168]  SetSaturation=off  Saturation=[0.6404,0.7127,0.8441,0.9214,0.9956,1.082,1.19,1.316,1.457;0.7,0.7698,0.8872,0.9466,0.9969,1.046,1.1,1.151,1.201]  LoadFlowParameters=[1 1000000000 0 0 0]  TsPowergui=0  TsBlock=-1  IterativeModel=Forward Euler  IterativeDiscreteModel=Trapezoidal non iterative  BusType=PV  Pref=P*1e6  Qref=0  Qmin=Qmin*1e6  Qmax=Qmax*1e6  PLF=0  QLF=0
      settings: AttributesFormatString=\n\n
  Pref : Constant
  Turbine & Regulators : Subsystem
  Vref : Constant
  A : PMIOPort  Side=Left
  B : PMIOPort  Port=2  Side=Left
  C : PMIOPort  Port=3  Side=Left
  m : Outport  VectorParamsAs1DForOutWhenUnconnected=off
  w : Outport  Port=2  VectorParamsAs1DForOutWhenUnconnected=off
  wires:
  Pref/1 -> Turbine & Regulators/2(Pref)
  Turbine & Regulators/2(Vf) -> Generator/2
  Generator/1 -> Turbine & Regulators/1(m)
  Vref/1 -> Turbine & Regulators/3(Vref)
  Turbine & Regulators/1(Pm) -> Generator/1
  Turbine & Regulators/3(Signals) -> Bus Selector/1, m/1
  Bus Selector/1 -> w/1  "<Rotor speed  wm  (pu)>"
  pss/1 -> Turbine & Regulators/4(d_Vstab)
  connections:
  A/RConn1 -- " MBASE MVA 400 kV-400 kV"/RConn1
  B/RConn1 -- " MBASE MVA 400 kV-400 kV"/RConn2
  C/RConn1 -- " MBASE MVA 400 kV-400 kV"/RConn3
  " MBASE MVA 400 kV-400 kV"/LConn1 -- Generator/RConn1
  " MBASE MVA 400 kV-400 kV"/LConn2 -- Generator/RConn2
  " MBASE MVA 400 kV-400 kV"/LConn3 -- Generator/RConn3

== system Nordic32_Lib/Trafo ==
  Three-Phase Parallel RLC Branch : powerlib/Elements/Three-Phase Parallel RLC Branch  Commented=on  LConnTagsString=A|B|C  RConnTagsString=A|B|C  BranchType=R  Resistance=1e6  Inductance=gen_Xt  Capacitance=1e-6  Measurements=None
      settings: SourceProductBaseCode=PS
  trafo : powerlib/Elements/Three-Phase Transformer (Two Windings)  Winding1Connection=Yg  Winding2Connection=Yg  CoreType=Three single-phase transformers  SetSaturation=off  Hysteresis=off  DataFile='hysteresis'  SetInitialFlux=off  Measurements=None  UNITS=pu  NominalPower="[ Sbase*1e6  fn]"  Winding1="[ratio*V1*1e3  1e-4   0  ]"  Winding2="[V2*1e3  1e-4  L2]"  Rm=1e6  Lm=1e6  L0=0.5  Saturation="[ 0,0  ;  0.005,1.2  ;  1.0,1.4 ]"  InitialFluxes=[ 0.8 , -0.8 , 0.7 ]  BreakLoop=off  DiscreteSolver=Trapezoidal iterative  DataType=off  TransfoNumber=0
  A : PMIOPort  Side=Left
  B : PMIOPort  Port=2  Side=Left
  C : PMIOPort  Port=3  Side=Left
  a : PMIOPort  Port=4  Side=Right
  b : PMIOPort  Port=5  Side=Right
  c : PMIOPort  Port=6  Side=Right
  connections:
  trafo/RConn2 -- Three-Phase Parallel RLC Branch/RConn2 -- b/RConn1
  trafo/LConn1 -- Three-Phase Parallel RLC Branch/LConn1 -- A/RConn1
  trafo/RConn1 -- Three-Phase Parallel RLC Branch/RConn1 -- a/RConn1
  trafo/LConn2 -- Three-Phase Parallel RLC Branch/LConn2 -- B/RConn1
  trafo/LConn3 -- Three-Phase Parallel RLC Branch/LConn3 -- C/RConn1
  trafo/RConn3 -- Three-Phase Parallel RLC Branch/RConn3 -- c/RConn1

== system Nordic32_Lib/Unwrap (step size 2*pi) ==
  u : Inport
  Delay : Delay  DelayLength=1
  Delay1 : Delay  DelayLength=1
  Demux : Demux  Outputs=2
  MATLAB Function : MATLAB Function  TreatAsAtomicUnit=on
  Mux : Mux  Inputs=3
  y : Outport
  wires:
  Mux/1 -> MATLAB Function/1(u)
  Delay/1 -> Mux/2
  u/1 -> Delay/1, Mux/1
  MATLAB Function/1(y) -> Demux/1
  Demux/1 -> y/1
  Demux/2 -> Delay1/1  "wrap count"
  Delay1/1 -> Mux/3
